simulink model "relay_action"  (R2021a)
settings: configuration reference "csro_code_gen_config" (kept outside this file)
settings Model: DataDictionary=motor_data.sldd  Creator=Litao  LastModifiedBy=Litao
settings ConfigSetRef: SourceName=csro_code_gen_config

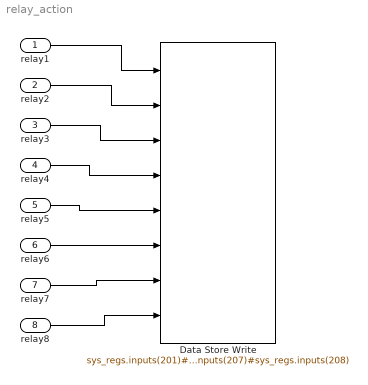
== system relay_action ==
  relay1 : Inport  OutDataTypeStr=int16
  relay2 : Inport  Port=2  OutDataTypeStr=int16
  relay3 : Inport  Port=3  OutDataTypeStr=int16
  relay4 : Inport  Port=4  OutDataTypeStr=int16
  relay5 : Inport  Port=5  OutDataTypeStr=int16
  relay6 : Inport  Port=6  OutDataTypeStr=int16
  relay7 : Inport  Port=7  OutDataTypeStr=int16
  relay8 : Inport  Port=8  OutDataTypeStr=int16
  Data Store Write : DataStoreWrite  DataStoreName=sys_regs  DataStoreElements=sys_regs.inputs(201)#sys_regs.inputs(202)#sys_regs.inputs(203)#sys_regs.inputs(204)#sys_regs.inputs(205)#sys_regs.inputs(206)#sys_regs.inputs(207)#sys_regs.inputs(208)  IndexOptions=Index vector (dialog)  Indices=1  OutputSizes=1
  wires:
  relay1/1 -> Data Store Write/1
  relay2/1 -> Data Store Write/2
  relay3/1 -> Data Store Write/3
  relay4/1 -> Data Store Write/4
  relay5/1 -> Data Store Write/5
  relay6/1 -> Data Store Write/6
  relay7/1 -> Data Store Write/7
  relay8/1 -> Data Store Write/8
